simulink model "AudioToBerOLD"  (R2014a)
settings: Solver=ode45  StartTime=0.0  StopTime=5.0  RelTol=1e-3
undefined symbols (not defined in the file or in its folder): rsgenpoly
libraries: commutil2 x2, commblkcod2 x2, commdigbbndfm2 x2, commchan3 x1, commsink2 x1
settings Model: Creator=HP  LastModifiedBy=HP

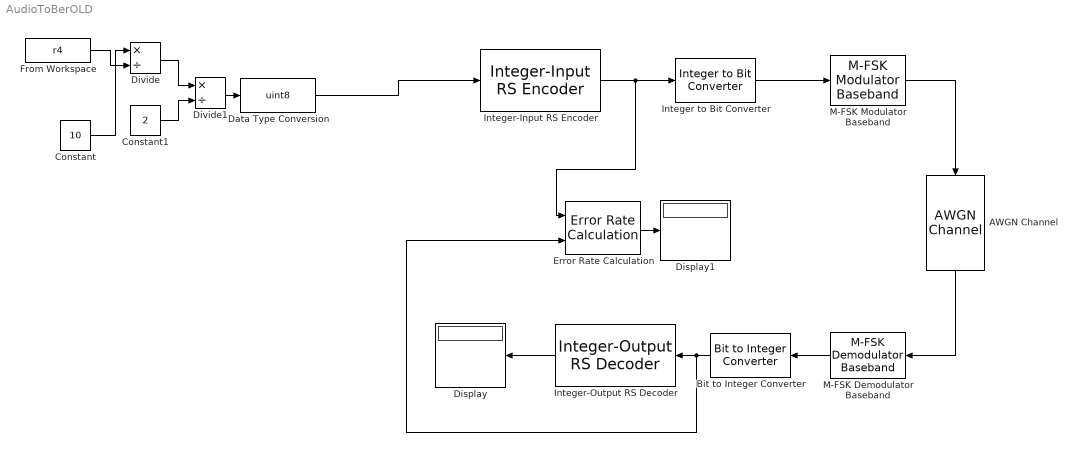
== system AudioToBerOLD ==
  AWGN Channel : commchan3/AWGN Channel  InputProcessing=Inherited (this choice will be removed - see release notes)  seed=67  noiseMode="Signal to noise ratio  (Eb/No)"  EbNodB=10  EsNodB=10  SNRdB=10  bitsPerSym=1  Ps=1  Tsym=1  variance=1
  Bit to Integer Converter : commutil2/Bit to Integer Converter  nbits=8  bitOrder=MSB first  signedOutputValues=Unsigned  outDtype=Inherit via internal rule  outDtypeSigned=Inherit via internal rule
  Constant : Constant  Value=10
  Constant1 : Constant  Value=2
  Data Type Conversion : DataTypeConversion  OutDataTypeStr=uint8  RndMeth=Round
  Display : Display
  Display1 : Display
  Divide : Product  Inputs=*/
  Divide1 : Product  Inputs=*/
  Error Rate Calculation : commsink2/Error Rate Calculation  N=0  st_delay=0  cp_mode=Entire frame  subframe=[]  PMode=Port  WsName=ErrorVec  RsMode2=off  stop=off  numErr=100  maxBits=1e6
  From Workspace : FromWorkspace  VariableName=r4  SampleTime=1
  Integer to Bit Converter : commutil2/Integer to Bit Converter  nbits=8  signedInputValues=Unsigned  bitOrder=MSB first  outDtype=Inherit via internal rule
  Integer-Input RS Encoder : commblkcod2/Integer-Input RS Encoder  n=255  k=155  specPrimPoly=off  prPoly=[1 0 1 1]  specGenPoly=on  genPoly=rsgenpoly(255,155)  specPuncture=off  punctVec=[ones(2,1); zeros(2,1)]
  Integer-Output RS Decoder : commblkcod2/Integer-Output RS Decoder  n=255  k=155  specPrimPoly=off  prPoly=[1 0 1 1]  specGenPoly=on  genPoly=rsgenpoly(255,155)  specPuncture=off  punctVec=[ones(2,1); zeros(2,1)]  specErasurePort=off  showNumErr=off
  M-FSK Demodulator Baseband : commdigbbndfm2/M-FSK Demodulator Baseband  M=256  OutType=Bit  Dec=Gray  freqSep=6  numSamp=17  RateOptions=Enforce single-rate processing  outDataType=double
  M-FSK Modulator Baseband : commdigbbndfm2/M-FSK Modulator Baseband  M=256  InType=Bit  Enc=Gray  freqSep=6  phaseType=Continuous  numSamp=17  RateOptions=Enforce single-rate processing  outDataType=double
  wires:
  Integer to Bit Converter/1 -> M-FSK Modulator Baseband/1
  M-FSK Modulator Baseband/1 -> AWGN Channel/1
  AWGN Channel/1 -> M-FSK Demodulator Baseband/1
  M-FSK Demodulator Baseband/1 -> Bit to Integer Converter/1
  Bit to Integer Converter/1 -> Error Rate Calculation/2, Integer-Output RS Decoder/1
  Integer-Output RS Decoder/1 -> Display/1
  Error Rate Calculation/1 -> Display1/1
  Integer-Input RS Encoder/1 -> Integer to Bit Converter/1, Error Rate Calculation/1
  From Workspace/1 -> Divide/2
  Constant/1 -> Divide/1
  Divide/1 -> Divide1/1
  Constant1/1 -> Divide1/2
  Divide1/1 -> Data Type Conversion/1
  Data Type Conversion/1 -> Integer-Input RS Encoder/1
